simulink model "final_part_4"  (Simulink 8.3)
settings: Solver=ode45  StartTime=0.0  StopTime=60  RelTol=1e-3
undefined symbols (not defined in the file or in its folder): drawMass, P
settings Model: Creator=beard  LastModifiedBy=jhl48
settings DataIOCC: LimitDataPoints=off
settings OptimizationCC: ExpressionDepthLimit=2147483647
settings DebuggingCC: SolverPrmCheckMsg=none  FcnCallInpInsideContextMsg=UseLocalSettings

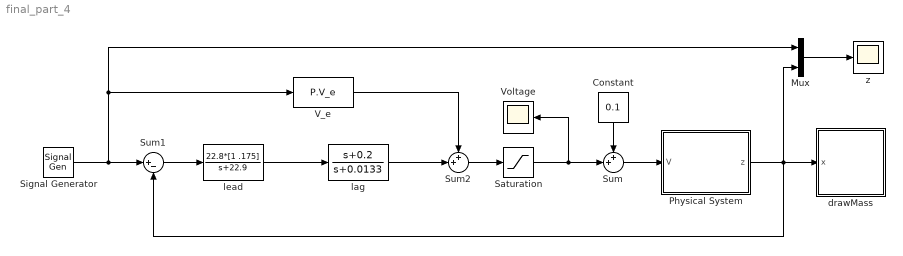
== system final_part_4 ==
  Constant : Constant  Value=0.1
  Mux : Mux  Inputs=2
  Physical System : Subsystem
  Saturation : Saturate  UpperLimit=P.V_max  LowerLimit=-P.V_max
  Signal Generator : SignalGenerator  WaveForm=square  Amplitude=0.5  Frequency=.025
  Sum : Sum  Inputs=++|
  Sum1 : Sum  Inputs=|+-
  Sum2 : Sum  Inputs=++|
  V_e : Fcn  Expr=P.V_e
  Voltage : Scope
      settings: TimeRange=60  YMin=-25  YMax=25  SaveName=ScopeData2
  drawMass : Subsystem
      mask init:
      | % drawing parameters
      | L = 5;
      | w = 1;
      | theta = 45*pi/180;
      mask Display: image(imread('tv.jpg'))
  lag : TransferFcn  Numerator=[1 0.2]  Denominator=[1 0.0133]
  lead : TransferFcn  Numerator=22.8*[1 .175]  Denominator=[1 22.9]
  z : Scope
      settings: TimeRange=60  YMin=-0.9  YMax=0.9
  wires:
  Signal Generator/1 -> V_e/1, Mux/1, Sum1/1
  Physical System/1(z) -> Sum1/2, Mux/2, drawMass/1(x)
  Saturation/1 -> Voltage/1, Sum/2
  Sum/1 -> Physical System/1(V)
  Constant/1 -> Sum/1
  Sum2/1 -> Saturation/1
  Mux/1 -> z/1
  lead/1 -> lag/1
  Sum1/1 -> lead/1
  lag/1 -> Sum2/2
  V_e/1 -> Sum2/1

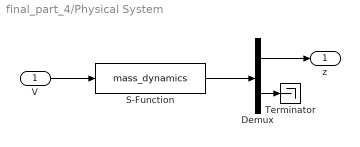
== system final_part_4/Physical System ==
  V : Inport
  Demux : Demux  Outputs=[1;3]
  S-Function : S-Function  FunctionName=mass_dynamics  Parameters=P  EnableBusSupport=off
  Terminator : Terminator
  z : Outport
  wires:
  Demux/1 -> z/1
  Demux/2 -> Terminator/1
  S-Function/1 -> Demux/1
  V/1 -> S-Function/1

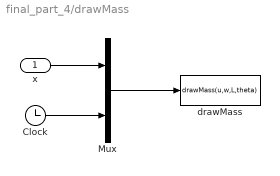
== system final_part_4/drawMass ==
  x : Inport
  Clock : Clock
  Mux : Mux  Inputs=2
  drawMass : MATLABFcn  MATLABFcn=drawMass(u,w,L,theta)  OutputDimensions=0  SampleTime=0.1
  wires:
  Mux/1 -> drawMass/1
  x/1 -> Mux/1
  Clock/1 -> Mux/2
